simulink model "dobgm1"  (Simulink 7.7)
settings: Solver=ode45  StartTime=0.0  StopTime=4  RelTol=1e-3
settings Model: Creator=potluri  LastModifiedBy=potluri

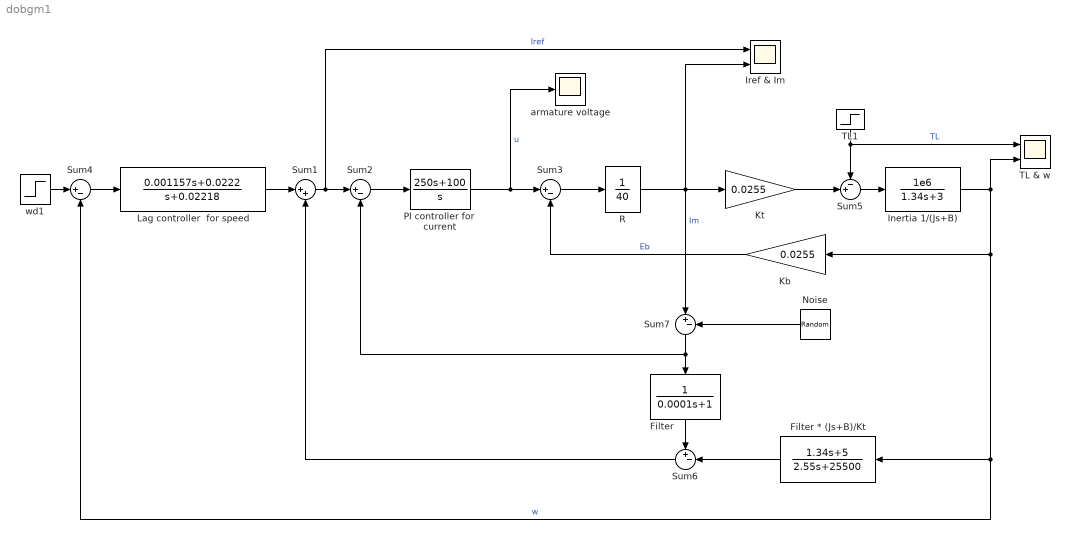
== system dobgm1 ==
  Filter : TransferFcn  Denominator=[0.0001 1]
  Filter * (Js+B)/Kt : TransferFcn  Numerator=[1.34 5]  Denominator=[2.55 25500]
  Inertia 1/(Js+B) : TransferFcn  Numerator=[1e6]  Denominator=[1.34 3]
  Iref & Im : Scope  NumInputPorts=2
      settings: YMin=0.6975~-5  YMax=0.715~5
  Kb : Gain  Gain=0.0255
  Kt : Gain  Gain=0.0255
  Lag controller  for speed : TransferFcn  Numerator=[0.001157 0.0222]  Denominator=[1 0.02218]
  Noise : RandomNumber  Variance=1e-2  SampleTime=0.002
  PI controller for  current : TransferFcn  Numerator=[250 100]  Denominator=[1 0]
  R : TransferFcn  Denominator=[40]
  Sum1 : Sum  Inputs=|++
  Sum{2..4,7} (4 alike) : Sum  Inputs=|+-
  Sum5 : Sum  Inputs=-+|
  Sum6 : Sum  Inputs=+-|
  TL & w : Scope  NumInputPorts=2
      settings: YMin=0.01615~99.2913  YMax=0.01785~99.2922  SaveName=ScopeData4
  TL1 : Step  After=0.017  SampleTime=0
  armature voltage : Scope
      settings: YMin=3  YMax=24  SaveName=ScopeData2
  wd1 : Step  Time=0  After=100  SampleTime=0
  wires:
  wd1/1 -> Sum4/1
  Sum1/1 -> Sum2/1, Iref & Im/1  "Iref"
  Sum2/1 -> PI controller for  current/1
  Sum3/1 -> R/1
  TL1/1 -> Sum5/1, TL & w/1  "TL"
  Sum5/1 -> Inertia 1/(Js+B)/1
  Inertia 1/(Js+B)/1 -> Kb/1, Filter * (Js+B)/Kt/1, Sum4/2, TL & w/2  "w"
  Kb/1 -> Sum3/2  "Eb"
  R/1 -> Kt/1, Iref & Im/2, Sum7/1  "Im"
  Kt/1 -> Sum5/2
  Filter/1 -> Sum6/1
  Filter * (Js+B)/Kt/1 -> Sum6/2
  PI controller for  current/1 -> Sum3/1, armature voltage/1  "u"
  Sum4/1 -> Lag controller  for speed/1
  Lag controller  for speed/1 -> Sum1/1
  Sum7/1 -> Filter/1, Sum2/2
  Noise/1 -> Sum7/2
  Sum6/1 -> Sum1/2
